simulink model "halfCarModel"  (R2016b)
settings: Solver=FixedStepAuto  StartTime=0.0  StopTime=5.0  FixedStep=.00001  RelTol=1e-3
settings Model: Creator=Devon  LastModifiedBy=Devon

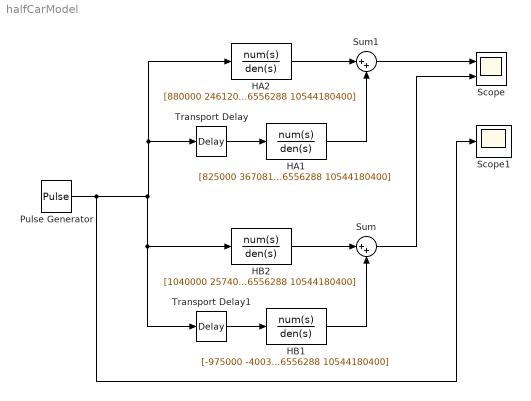
== system halfCarModel ==
  HA1 : TransferFcn  Numerator=[825000 36708150 433278144 5272090200]  Denominator=[275000 4324500 130604235 866556288 10544180400]
  HA2 : TransferFcn  Numerator=[880000 24612000 433278144 5272090200]  Denominator=[275000 4324500 130604235 866556288 10544180400]
  HB1 : TransferFcn  Numerator=[-975000 -40035450 -333290880 -4055454000]  Denominator=[275000 4324500 130604235 866556288 10544180400]
  HB2 : TransferFcn  Numerator=[1040000 25740000 333290880 4055454000]  Denominator=[275000 4324500 130604235 866556288 10544180400]
  Pulse Generator : DiscretePulseGenerator  PulseType=Time based  Amplitude=.02  Period=10  PulseWidth=.005
  Scope : Scope  NumInputPorts=2
  Scope1 : Scope
  Sum : Sum  Inputs=|++
  Sum1 : Sum  Inputs=|++
  Transport Delay : TransportDelay
  Transport Delay1 : TransportDelay
  wires:
  Pulse Generator/1 -> Scope1/1, HB2/1, Transport Delay1/1, Transport Delay/1, HA2/1
  Transport Delay1/1 -> HB1/1
  HB2/1 -> Sum/1
  HB1/1 -> Sum/2
  HA2/1 -> Sum1/1
  HA1/1 -> Sum1/2
  Sum1/1 -> Scope/1
  Sum/1 -> Scope/2
  Transport Delay/1 -> HA1/1
